simulink model "Actuator_FaultInjection_Model"  (R2026a)
settings: Solver=ode45  StopTime=20  MaxStep=1e-4
values from neighbouring files (symbols this model uses):
  Bnom = 0.0004    [actuator_params.mat]    (also in build_model.m)
  J = 0.0008    [actuator_params.mat]    (also in build_model.m)
  Ke = 0.05    [actuator_params.mat]    (also in build_model.m)
  Kt = 0.05    [actuator_params.mat]    (also in build_model.m)
  L = 0.003    [actuator_params.mat]    (also in build_model.m)
  Rnom = 0.8    [actuator_params.mat]    (also in build_model.m)
  Tload = 0.02    [actuator_params.mat]    (also in build_model.m)
  Vin_amp = 24    [actuator_params.mat]    (also in build_model.m)
settings Model: Creator=Nirmal patil  LastModifiedBy=Nirmal patil

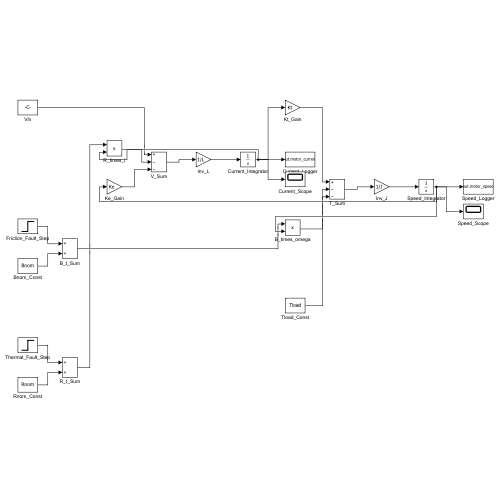
[thumbnail: Simulink's stored preview of the top-level diagram]
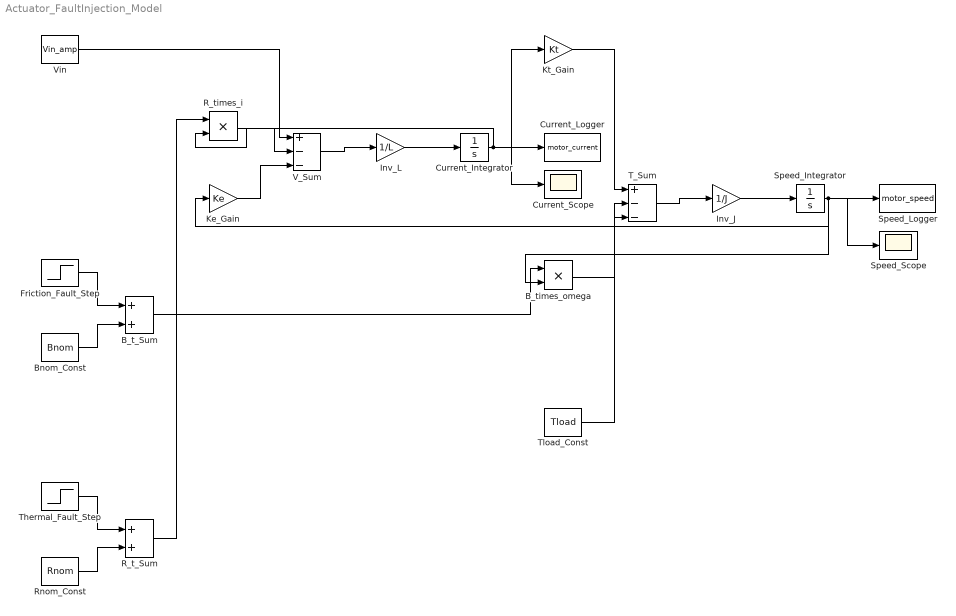
== system Actuator_FaultInjection_Model ==
  B_t_Sum : Sum
  B_times_omega : Product
  Bnom_Const : Constant  Value=Bnom
  Current_Integrator : Integrator
  Current_Logger : ToWorkspace  VariableName=motor_current  SaveFormat=Timeseries  SampleTime=-1
  Current_Scope : Scope
  Friction_Fault_Step : Step  Time=8  FinalValue=0.0006  SampleTime=0
  Inv_J : Gain  Gain=1/J
  Inv_L : Gain  Gain=1/L
  Ke_Gain : Gain  Gain=Ke
  Kt_Gain : Gain  Gain=Kt
  R_t_Sum : Sum
  R_times_i : Product
  Rnom_Const : Constant  Value=Rnom
  Speed_Integrator : Integrator
  Speed_Logger : ToWorkspace  VariableName=motor_speed  SaveFormat=Timeseries  SampleTime=-1
  Speed_Scope : Scope
  T_Sum : Sum  Inputs=+--
  Thermal_Fault_Step : Step  Time=14  FinalValue=0.64  SampleTime=0
  Tload_Const : Constant  Value=Tload
  V_Sum : Sum  Inputs=+--
  Vin : Constant  Value=Vin_amp
  wires:
  Friction_Fault_Step/1 -> B_t_Sum/1
  Bnom_Const/1 -> B_t_Sum/2
  Thermal_Fault_Step/1 -> R_t_Sum/1
  Rnom_Const/1 -> R_t_Sum/2
  R_t_Sum/1 -> R_times_i/1
  Current_Integrator/1 -> R_times_i/2, Kt_Gain/1, Current_Logger/1, Current_Scope/1
  Speed_Integrator/1 -> Ke_Gain/1, B_times_omega/2, Speed_Logger/1, Speed_Scope/1
  Vin/1 -> V_Sum/1
  R_times_i/1 -> V_Sum/2
  Ke_Gain/1 -> V_Sum/3
  V_Sum/1 -> Inv_L/1
  Inv_L/1 -> Current_Integrator/1
  B_t_Sum/1 -> B_times_omega/1
  Kt_Gain/1 -> T_Sum/1
  B_times_omega/1 -> T_Sum/2
  Tload_Const/1 -> T_Sum/3
  T_Sum/1 -> Inv_J/1
  Inv_J/1 -> Speed_Integrator/1
